simulink model "CyberResilient_ActiveSuspension"  (R2024b)
settings: Solver=ode4  StartTime=0.0  StopTime=10  FixedStep=0.001  RelTol=1e-3
settings Model: Creator=sange  LastModifiedBy=sange
settings DataIOCC: SaveFormat=StructureWithTime  OutputSaveName=sim_yout

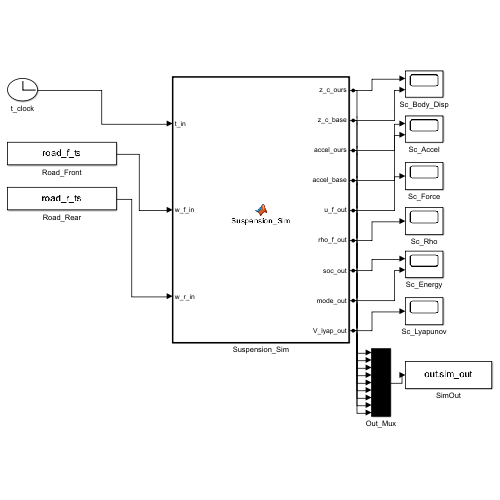
[thumbnail: Simulink's stored preview of the top-level diagram]
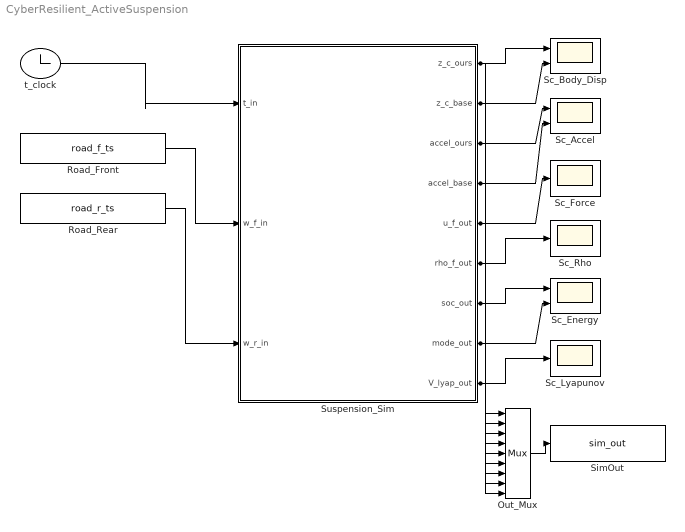
== system CyberResilient_ActiveSuspension ==
  Out_Mux : Mux  Inputs=9
  Road_Front : FromWorkspace  VariableName=road_f_ts
  Road_Rear : FromWorkspace  VariableName=road_r_ts
  Sc_Accel : Scope  NumInputPorts=2
  Sc_Body_Disp : Scope  NumInputPorts=2
  Sc_Energy : Scope  NumInputPorts=2
  Sc_Force : Scope
  Sc_Lyapunov : Scope
  Sc_Rho : Scope
  SimOut : ToWorkspace  VariableName=sim_out  SaveFormat=Structure With Time  SampleTime=-1
  Suspension_Sim : MATLAB Function  TreatAsAtomicUnit=on
  t_clock : Clock
  wires:
  t_clock/1 -> Suspension_Sim/1(t_in)
  Road_Front/1 -> Suspension_Sim/2(w_f_in)
  Road_Rear/1 -> Suspension_Sim/3(w_r_in)
  Suspension_Sim/1(z_c_ours) -> Sc_Body_Disp/1, Out_Mux/1
  Suspension_Sim/2(z_c_base) -> Sc_Body_Disp/2, Out_Mux/2
  Suspension_Sim/3(accel_ours) -> Sc_Accel/1, Out_Mux/3
  Suspension_Sim/4(accel_base) -> Sc_Accel/2, Out_Mux/4
  Suspension_Sim/5(u_f_out) -> Sc_Force/1, Out_Mux/5
  Suspension_Sim/6(rho_f_out) -> Sc_Rho/1, Out_Mux/6
  Suspension_Sim/7(soc_out) -> Sc_Energy/1, Out_Mux/7
  Suspension_Sim/8(mode_out) -> Sc_Energy/2, Out_Mux/8
  Suspension_Sim/9(V_lyap_out) -> Sc_Lyapunov/1, Out_Mux/9
  Out_Mux/1 -> SimOut/1

== matlab function CyberResilient_ActiveSuspension/Suspension_Sim ==
  data: t_in input; z_c_ours output; w_f_in input; w_r_in input; z_c_base output; accel_ours output; accel_base output; u_f_out output; rho_f_out output; soc_out output; mode_out output; V_lyap_out output
function [z_c_ours, z_c_base, accel_ours, accel_base, u_f_out, rho_f_out, soc_out, mode_out, V_lyap_out] = Suspension_Sim(t_in, w_f_in, w_r_in)
% Cyber-Resilient LPV-Adaptive Active Suspension — Simulink MATLAB Function Block
% All parameters hardcoded. State maintained via persistent variables.
% Automatically re-initialises when t_in resets to 0 (new simulation run).

persistent st_ours st_base bat_soc lc_il lc_vc
persistent rho_f_p rdot_filt mets_last mets_first

% ---- VEHICLE PARAMETERS (hardcoded numeric literals) ----
ms    = 730.0000;  I_phi = 1222.0000;
a     = 1.1000;  b     = 1.5000;
mu_f  = 45.0000;  mu_r  = 45.0000;
ks_f  = 18000.00; ks_r  = 22000.00;
cs_f  = 1200.00;  cs_r  = 1200.00;
kt_f  = 190000.00; kt_r  = 190000.00;
k_em  = 15.0000; i_d   = 20.0000;  p_pole = 8;
whr   = 0.3000; v_ms  = 20.0000;
C_e   = 1500.0000; eta_r = 0.6500;  K_v    = 50.0000;
smax  = 0.080000; u_max = 6000.0000;  k_bs   = 1.000000e+07;
Lf    = 0.010000; Cf    = 0.00470000;  Rl     = 10.0000;
sig_m = 0.1000;
dt = 0.001; w_max = 0.05; ema_a = 0.05; eta_act = 0.85; cap_j = 50000;

% ---- CONTROLLER GAINS (computed from CARE, substituted as literals) ----
Ks  = [2591.260282 2545.019204 -4409.593492 -22.6009354];
Kr  = [1339.079606 6792.410633 -15288.11257 39.41237591];
Krd = [0 500 0 0];
Pl  = [55514.66518 1292.584418 51939.7711 21.505047;1292.584418 1223.579227 -1867.584611 16.21273818;51939.7711 -1867.584611 68939.36182 -1.11842938;21.505047 16.21273818 -1.11842938 2.749362062];
Kbf = [-12000 5500 8000 0 -3500 1800 2200 0];
Kbr = [-12000 -5500 0 8000 -3500 -1800 0 2200];

% ---- INITIALISE on first call OR when t_in resets to 0 ----
if isempty(st_ours) || (t_in < 5e-4)
    st_ours = zeros(8,1);  st_base = zeros(8,1);
    bat_soc = 0.5;  lc_il = 0;  lc_vc = 0;
    rho_f_p = 0;   rdot_filt = 0;
    mets_last = zeros(8,1);  mets_first = true;
end

wf = w_f_in;  wr = w_r_in;

% ==== BASE PAPER: Fixed H-infinity controller ====
uf_b = max(-u_max, min(u_max, -Kbf * st_base));
ur_b = max(-u_max, min(u_max, -Kbr * st_base));
[st_base, dx_b] = rk4_hc(t_in, st_base, uf_b, ur_b, wf, wr, ...
    ms,I_phi,a,b,mu_f,mu_r,ks_f,ks_r,cs_f,cs_r,kt_f,kt_r,k_em,i_d,p_pole,whr,v_ms,smax,k_bs,dt);

% ==== OUR PROJECT: LPV + UKF + TD3 + METS ====
% Step A: METS Network Filter
if mets_first
    mets_last = st_ours;  mets_first = false;  net = st_ours;
else
    em = st_ours - mets_last;
    ne = sqrt(em(1)^2+em(2)^2+em(3)^2+em(4)^2+em(5)^2+em(6)^2+em(7)^2+em(8)^2);
    nx = sqrt(st_ours(1)^2+st_ours(2)^2+st_ours(3)^2+st_ours(4)^2+st_ours(5)^2+st_ours(6)^2+st_ours(7)^2+st_ours(8)^2);
    if ne > sig_m * nx;  mets_last = st_ours;  net = st_ours;
    else;                                       net = mets_last;  end
end

% Step B: UKF Road Severity Estimator (simplified algebraic)
rho_f     = min(1.0, max(0.0, abs(st_ours(1) - a*st_ours(2) - st_ours(3)) / w_max));
rdot_filt = ema_a * ((rho_f - rho_f_p) / dt) + (1.0 - ema_a) * rdot_filt;
rho_dot   = rdot_filt;  rho_f_p = rho_f;

% Step C: TD3 Heuristic Energy Agent
if rho_f > 0.7 || rho_dot > 0.5
    if bat_soc < 0.02;  mf = 1;  else;  mf = 0;  end
elseif rho_f > 0.3
    if bat_soc < 0.25;  mf = 1;  else;  mf = 0;  end
else
    mf = 1;  % Smooth road — harvest energy
end

% Step D: LPV Controller — Quarter-Car State Mapping
zsf  = net(1) - a*net(2);   zsfd = net(5) - a*net(6);
qcf  = [zsf - net(3); zsfd; 0; net(7)];
zsr  = net(1) + b*net(2);   zsrd = net(5) + b*net(6);
qcr  = [zsr - net(4); zsrd; 0; net(8)];
ffl  = 0.2 * u_max;
if mf == 1  % ECO: regenerative damping
    ufo = -C_e * qcf(2);  uro = -C_e * qcr(2);
else        % COMFORT: LPV active control
    Kf  = (1.0 - rho_f) * Ks + rho_f * Kr;
    ufo = (-Kf * qcf) + max(-ffl, min(ffl, -Krd * max(0, rho_dot) * qcf));
    uro = (-Kf * qcr) + max(-ffl, min(ffl, -Krd * max(0, rho_dot) * qcr));
end
ufo = max(-u_max, min(u_max, ufo));
uro = max(-u_max, min(u_max, uro));

% Step E: RK4 Physics Integration
[st_ours, dx_o] = rk4_hc(t_in, st_ours, ufo, uro, wf, wr, ...
    ms,I_phi,a,b,mu_f,mu_r,ks_f,ks_r,cs_f,cs_r,kt_f,kt_r,k_em,i_d,p_pole,whr,v_ms,smax,k_bs,dt);

% Step F: Energy Harvesting with LC Power Electronics Filter
vrf = (st_ours(5) - a*st_ours(6)) - st_ours(7);  % Front suspension rel. velocity
if mf == 1  % ECO mode: harvest
    vrect = abs(K_v * vrf);
    di_L  = (vrect - lc_vc) / Lf;
    dv_C  = (lc_il - lc_vc / Rl) / Cf;
    lc_il = min(max(lc_il + di_L * dt, 0), 100);  % Clamped for numerical stability
    lc_vc = min(max(lc_vc + dv_C * dt, 0), 500);
    harv  = (lc_vc^2 / Rl) * eta_r * dt;
    bat_soc = min(1.0, bat_soc + harv / cap_j);
else  % COMFORT mode: consume battery
    bat_soc = max(0.0, bat_soc - abs(ufo * vrf) / eta_act * dt / cap_j);
    lc_il = lc_il * 0.99;  lc_vc = lc_vc * 0.99;  % LC filter decays
end

% Step G: Lyapunov Stability Monitor — V(x) = x_qc' * P * x_qc
xq  = [st_ours(1)-a*st_ours(2)-st_ours(3); st_ours(5)-a*st_ours(6); 0; st_ours(7)];
V_x = xq' * Pl * xq;

% ---- OUTPUTS ----
z_c_ours   = st_ours(1);  z_c_base   = st_base(1);
accel_ours = dx_o(5);     accel_base = dx_b(5);
u_f_out    = ufo;         rho_f_out  = rho_f;
soc_out    = bat_soc;     mode_out   = double(mf);
V_lyap_out = V_x;
end  % Suspension_Sim

% ===== LOCAL: 4th-Order Runge-Kutta =====
function [ns, k1] = rk4_hc(t, x, uf, ur, wf, wr, ms, Ip, a, b, muf, mur, ksf, ksr, csf, csr, ktf, ktr, kem, id, pp, whr, vms, sm, kbs, dt)
    k1 = hc_ode(t,       x,         uf,ur,wf,wr,ms,Ip,a,b,muf,mur,ksf,ksr,csf,csr,ktf,ktr,kem,id,pp,whr,vms,sm,kbs);
    k2 = hc_ode(t+dt/2,  x+k1*dt/2, uf,ur,wf,wr,ms,Ip,a,b,muf,mur,ksf,ksr,csf,csr,ktf,ktr,kem,id,pp,whr,vms,sm,kbs);
    k3 = hc_ode(t+dt/2,  x+k2*dt/2, uf,ur,wf,wr,ms,Ip,a,b,muf,mur,ksf,ksr,csf,csr,ktf,ktr,kem,id,pp,whr,vms,sm,kbs);
    k4 = hc_ode(t+dt,    x+k3*dt,   uf,ur,wf,wr,ms,Ip,a,b,muf,mur,ksf,ksr,csf,csr,ktf,ktr,kem,id,pp,whr,vms,sm,kbs);
    ns  = x + (dt / 6) * (k1 + 2*k2 + 2*k3 + k4);
end

% ===== LOCAL: 4-DOF Half-Car ODE =====
function dx = hc_ode(t, x, uf, ur, wf, wr, ms, Ip, a, b, muf, mur, ksf, ksr, csf, csr, ktf, ktr, kem, id, pp, whr, vms, sm, kbs)
    z_c=x(1); th=x(2); zuf=x(3); zur=x(4); zcd=x(5); thd=x(6); zufd=x(7); zurd=x(8);
    zsf=z_c-a*th;  zsr=z_c+b*th;  zsfd=zcd-a*thd;  zsrd=zcd+b*thd;
    dsf=zsf-zuf;   dsr=zsr-zur;   dtf=zuf-wf;      dtr=zur-wr;
    vrf=zsfd-zufd; vrr=zsrd-zurd;
    if     dsf >  sm;  fb_f = kbs*(dsf-sm)^3;
    elseif dsf < -sm;  fb_f = kbs*(dsf+sm)^3;
    else;              fb_f = 0;  end
    if     dsr >  sm;  fb_r = kbs*(dsr-sm)^3;
    elseif dsr < -sm;  fb_r = kbs*(dsr+sm)^3;
    else;              fb_r = 0;  end
    fiwm = kem * id * sin(pp * (vms/whr) * t);
    Fsf  = ksf*dsf + csf*vrf + fb_f - uf;
    Fsr  = ksr*dsr + csr*vrr + fb_r - ur;
    dx = [zcd; thd; zufd; zurd; ...
          -(Fsf+Fsr)/ms; (a*Fsf-b*Fsr)/Ip; ...
          (Fsf - ktf*dtf + fiwm)/muf; (Fsr - ktr*dtr + fiwm)/mur];
end
